simulink model "testtemp"  (Simulink 6.2)
settings: Solver=ode4  SolverMode=SingleTasking  StartTime=0  StopTime=0  MaxStep=10  RelTol=1e-3  AbsTol=1e-3
undefined symbols (not defined in the file or in its folder): d, n, pdelay, tgain, velreconsw
(part 1 of 3)
settings Model: Creator=jacobs  LastModifiedBy=jacobs  ExtModeAutoUpdateStatusClock=off
settings DataIOCC: LimitDataPoints=off  SaveOutput=off  SaveTime=off
settings OptimizationCC: BlockReduction=off  BooleanDataType=off
settings HardwareCC: TargetUnknown=on
settings STFCustomTargetCC: TargetFcnLib=ansi_tfl_tmw.mat  GenFloatMathFcnCalls=ANSI_C  ModelReferenceCompliant=off  SystemTargetFile=grt.tlc

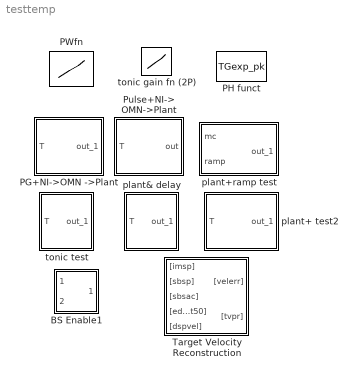
== system testtemp ==
  BS Enable1 : Subsystem
      mask Display: disp('FS\nEnab')
  PG+NI->OMN ->Plant : Subsystem
      mask Display: disp('PG+NI\n->OMN\n->Plant')
  PH funct : MATLABFcn  MATLABFcn=TGexp_pk
      mask Display: disp('Tonic\nGain')
  PWfn : Lookup  Orientation=down  InputValues=[ 0, 0.05:5, 5:10, 10:50 ]  OutputValues="[ 0, (0.05:5)*0+15,  (5:10)*1+10,  (10:50)*2]"  SaturateOnIntegerOverflow=on
  Pulse+NI-> OMN->Plant : Subsystem
      mask Display: disp('Pulse+NI\n->OMN\n->Plant')
  Target Velocity Reconstruction : Subsystem
      mask Display: disp('Target\nVelocity\nReconstruction')
  plant& delay : Subsystem
      mask Display: disp('plant &\ndelay')
  plant+ test2 : Subsystem
      mask Display: disp('PG->delay\n->plant')
  plant+ramp test : Subsystem
      mask Display: disp('plant+ramp\ntest')
  tonic gain fn (2P) : Lookup  InputValues=[ 0:90, 90:120 ]  OutputValues=[ (0:90)*( -.0039)+5.6, (90:120)*(-.0326)+8.18 ]  SaturateOnIntegerOverflow=on
  tonic test : Subsystem
      mask Display: disp('tonic\ntest')

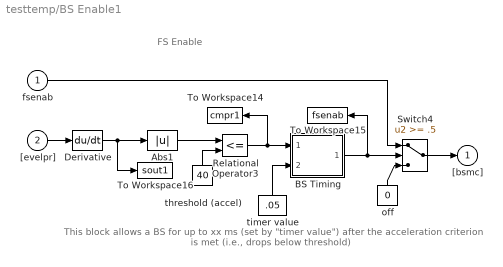
== system testtemp/BS Enable1 ==
  note: FS Enable
  note: This block allows a BS for up to xx ms (set by "timer value")
      | after the acceleration criterion is met (i.e., drops below threshold)
  fsenab : Inport  Port=1  LatchInput=off
  "[evelpr]" : Inport  Port=2  LatchInput=off
  Abs1 : Abs  SaturateOnIntegerOverflow=on
  BS Timing : Subsystem
      mask Display: disp('FS\nEnable\nTiming')
  Derivative : Derivative
      mask Display: disp('s')
  Relational Operator3 : RelationalOperator  Operator=<=  InputSameDT=on
  Switch4 : Switch  Threshold=.5  SaturateOnIntegerOverflow=on  InputSameDT=on
  To Workspace14 : ToWorkspace  VariableName=cmpr1  SaveFormat=Array
      settings: MaxDataPoints=10000
      mask Type: imsw1in
  To Workspace15 : ToWorkspace  VariableName=fsenab  SaveFormat=Array
      settings: MaxDataPoints=10000
      mask Type: imsw1in
  To Workspace16 : ToWorkspace  VariableName=sout1  SaveFormat=Array
      settings: MaxDataPoints=10000
      mask Type: imsw1in
  off : Constant  Orientation=up  Value=0
  threshold (accel) : Constant  Orientation=up  Value=40
  timer value : Constant  Orientation=up  Value=.05
  "[bsmc]" : Outport  InitialOutput=0
  wires:
  Relational Operator3/1 -> To Workspace14/1, BS Timing/1(From  <= [cmpr])
  Derivative/1 -> To Workspace16/1, Abs1/1
  Abs1/1 -> Relational Operator3/1
  BS Timing/1("[bsenab]") -> To Workspace15/1, Switch4/2
  "[evelpr]"/1 -> Derivative/1
  off/1 -> Switch4/3
  threshold (accel)/1 -> Relational Operator3/2
  fsenab/1 -> Switch4/1
  Switch4/1 -> "[bsmc]"/1
  timer value/1 -> BS Timing/2(timer dur)

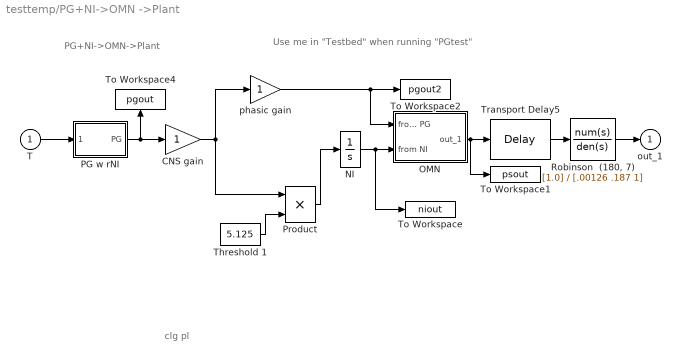
== system testtemp/PG+NI->OMN ->Plant ==
  note: clg
      | pl
  note: Use me in "Testbed" when running "PGtest"
  note: PG+NI->OMN->Plant
  T : Inport  Port=1  LatchInput=off
  CNS gain : Gain  SaturateOnIntegerOverflow=on
  NI : Integrator
  OMN : Subsystem
      mask Display: disp('<--"phasic"\nOMN\n<--"tonic"   ')
  PG w rNI : Subsystem
      mask Display: disp('PG rNI\n(2P)')
  Product : Product  SaturateOnIntegerOverflow=on  RndMeth=Zero  InputSameDT=on
  "Robinson  (180, 7)" : TransferFcn  Numerator=[1.0]  Denominator=[.00126 .187 1]
      mask Display: disp('2-pole')
  Threshold 1 : Constant  Value=5.125
  To Workspace : ToWorkspace  VariableName=niout  SaveFormat=Array
      settings: MaxDataPoints=10000
  To Workspace1 : ToWorkspace  VariableName=psout  SaveFormat=Array
      settings: MaxDataPoints=10000
  To Workspace2 : ToWorkspace  VariableName=pgout2  SaveFormat=Array
      settings: MaxDataPoints=10000
  To Workspace4 : ToWorkspace  VariableName=pgout  SaveFormat=Array
      settings: Orientation=up  MaxDataPoints=10000
  Transport Delay5 : TransportDelay  DelayTime=0.001
      mask Display: disp('"pdelay"\n(msec)')
  phasic gain : Gain  SaturateOnIntegerOverflow=on
  out_1 : Outport  InitialOutput=0
  wires:
  Threshold 1/1 -> Product/2
  PG w rNI/1(PG) -> CNS gain/1, To Workspace4/1
  Transport Delay5/1 -> "Robinson  (180, 7)"/1
  Product/1 -> NI/1
  "Robinson  (180, 7)"/1 -> out_1/1
  NI/1 -> OMN/2(from NI), To Workspace/1
  phasic gain/1 -> To Workspace2/1, OMN/1(from PG)
  OMN/1(out_1) -> Transport Delay5/1, To Workspace1/1
  CNS gain/1 -> phasic gain/1, Product/1
  T/1 -> PG w rNI/1(mcsprd)

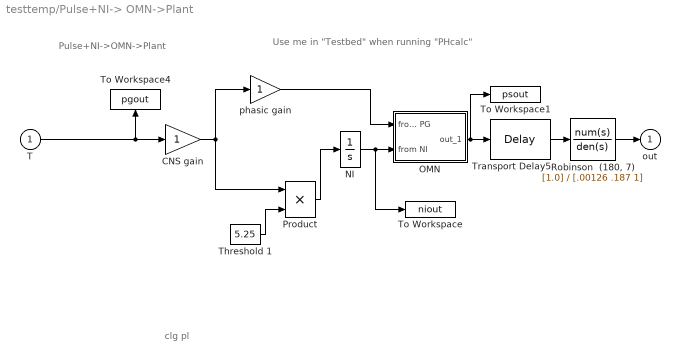
== system testtemp/Pulse+NI-> OMN->Plant ==
  note: clg
      | pl
  note: Use me in "Testbed" when running "PHcalc"
  note: Pulse+NI->OMN->Plant
  T : Inport  Port=1  LatchInput=off
  CNS gain : Gain  SaturateOnIntegerOverflow=on
  NI : Integrator
  OMN : Subsystem
      mask Display: disp('<--"phasic"\nOMN\n<--"tonic"   ')
  Product : Product  SaturateOnIntegerOverflow=on  RndMeth=Zero  InputSameDT=on
  "Robinson  (180, 7)" : TransferFcn  Numerator=[1.0]  Denominator=[.00126 .187 1]
      mask Display: disp('2-pole')
  Threshold 1 : Constant  Value=5.25
  To Workspace : ToWorkspace  VariableName=niout  SaveFormat=Array
      settings: MaxDataPoints=10000
  To Workspace1 : ToWorkspace  VariableName=psout  SaveFormat=Array
      settings: MaxDataPoints=10000
  To Workspace4 : ToWorkspace  VariableName=pgout  SaveFormat=Array
      settings: Orientation=up  MaxDataPoints=10000
  Transport Delay5 : TransportDelay  DelayTime=0.001
      mask Display: disp('"pdelay"\n(msec)')
  phasic gain : Gain  SaturateOnIntegerOverflow=on
  out : Outport  InitialOutput=0
  wires:
  Threshold 1/1 -> Product/2
  T/1 -> CNS gain/1, To Workspace4/1
  Transport Delay5/1 -> "Robinson  (180, 7)"/1
  Product/1 -> NI/1
  "Robinson  (180, 7)"/1 -> out/1
  NI/1 -> OMN/2(from NI), To Workspace/1
  phasic gain/1 -> OMN/1(from PG)
  OMN/1(out_1) -> Transport Delay5/1, To Workspace1/1
  CNS gain/1 -> phasic gain/1, Product/1

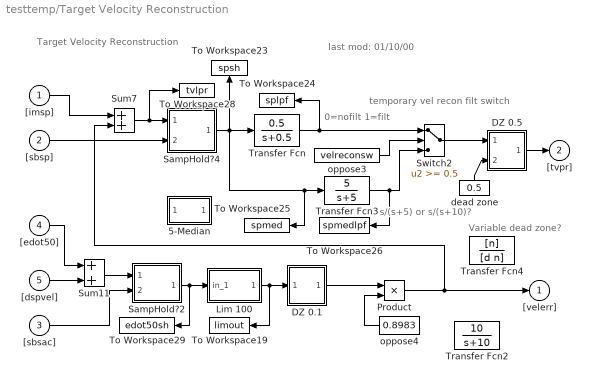
== system testtemp/Target Velocity Reconstruction ==
  note: last mod:
      | 01/10/00
  note: Target Velocity Reconstruction
  note: temporary
      | vel recon
      | filt switch
  note: 0=nofilt
      | 1=filt
  note: s/(s+5) or
      | s/(s+10)?
  note: Variable dead zone?
  "[imsp]" : Inport  Port=1  LatchInput=off
  "[sbsp]" : Inport  Port=2  LatchInput=off
  "[sbsac]" : Inport  Port=3  LatchInput=off
  "[edot50]" : Inport  Port=4  LatchInput=off
  "[dspvel]" : Inport  Port=5  LatchInput=off
  5-Median : Subsystem
      mask Display: disp('5-Med')
  DZ 0.1 : Subsystem
      mask Display: disp('Dead\nZone')
  DZ 0.5 : Subsystem
      mask Display: disp('Dead\nZone')
  Lim 100 : Subsystem
      mask Display: disp('Limiter')
  Product : Product  SaturateOnIntegerOverflow=on  RndMeth=Zero  InputSameDT=on
  SampHold?2 : Subsystem
      mask Display: disp('S=H\nH=L')
  SampHold?4 : Subsystem
      mask Display: disp('S=H\nH=L')
  Sum11 : Sum  SaturateOnIntegerOverflow=on  InputSameDT=on
  Sum7 : Sum  SaturateOnIntegerOverflow=on  InputSameDT=on
  Switch2 : Switch  Threshold=0.5  SaturateOnIntegerOverflow=on  InputSameDT=on
  To Workspace19 : ToWorkspace  VariableName=limout  SaveFormat=Array
      settings: MaxDataPoints=10000
  To Workspace23 : ToWorkspace  VariableName=spsh  SaveFormat=Array
      settings: Orientation=up  MaxDataPoints=10000
  To Workspace24 : ToWorkspace  VariableName=splpf  SaveFormat=Array
      settings: MaxDataPoints=10000
  To Workspace25 : ToWorkspace  VariableName=spmed  SaveFormat=Array
      settings: MaxDataPoints=10000
  To Workspace26 : ToWorkspace  VariableName=spmedlpf  SaveFormat=Array
      settings: MaxDataPoints=10000
  To Workspace28 : ToWorkspace  VariableName=tvlpr  SaveFormat=Array
      settings: MaxDataPoints=10000
  To Workspace29 : ToWorkspace  VariableName=edot50sh  SaveFormat=Array
      settings: MaxDataPoints=10000
  Transfer Fcn : TransferFcn  Numerator=[0.5]  Denominator=[1 0.5]
  Transfer Fcn2 : TransferFcn  Numerator=[10]  Denominator=[1 10]
  Transfer Fcn3 : TransferFcn  Numerator=[5]  Denominator=[1 5]
  Transfer Fcn4 : TransferFcn  Numerator=[n]  Denominator=[d n]
  dead zone : Constant  Orientation=up  Value=0.5
  oppose3 : Constant  Value=velreconsw
  oppose4 : Constant  Orientation=left  Value=0.8983
  "[velerr]" : Outport  InitialOutput=0
  "[tvpr]" : Outport  Port=2  InitialOutput=0
  wires:
  "[sbsp]"/1 -> SampHold?4/2(S/H?)
  SampHold?4/1(output) -> Transfer Fcn/1, To Workspace23/1, To Workspace25/1, Transfer Fcn3/1
  "[imsp]"/1 -> Sum7/1
  Sum7/1 -> SampHold?4/1(Input), To Workspace28/1
  Transfer Fcn/1 -> To Workspace24/1, Switch2/1
  oppose3/1 -> Switch2/2
  Switch2/1 -> DZ 0.5/1(in_1)
  "[sbsac]"/1 -> SampHold?2/2(S/H?)
  "[dspvel]"/1 -> Sum11/2
  "[edot50]"/1 -> Sum11/1
  Sum11/1 -> SampHold?2/1(Input)
  Lim 100/1(out_1) -> To Workspace19/1, DZ 0.1/1(in_1)
  SampHold?2/1(output) -> To Workspace29/1, Lim 100/1(in_1)
  DZ 0.1/1(out_1) -> Product/1
  Product/1 -> Sum7/2, "[velerr]"/1
  oppose4/1 -> Product/2
  DZ 0.5/1(out_1) -> "[tvpr]"/1
  dead zone/1 -> DZ 0.5/2(in_2)
  Transfer Fcn3/1 -> Switch2/3, To Workspace26/1

== system testtemp/plant& delay ==
  note: clg
      | pl
  note: Use me in "Testbed" when running "PHcalc"
  T : Inport  Port=1  LatchInput=off
  "Robinson  (180, 7)" : TransferFcn  Numerator=[1.0]  Denominator=[.00126 .187 1]
      mask Display: disp('2-pole')
  Transport Delay5 : TransportDelay  DelayTime=pdelay
      mask Display: disp('"pdelay"\n(ms)')
  out_1 : Outport  InitialOutput=0
  wires:
  "Robinson  (180, 7)"/1 -> out_1/1
  T/1 -> Transport Delay5/1
  Transport Delay5/1 -> "Robinson  (180, 7)"/1

== system testtemp/plant+ test2 ==
  note: clg
      | pl
  note: PG->delay->Plant
  T : Inport  Port=1  LatchInput=off
  PG w rNI : Subsystem
      mask Display: disp('PG rNI\n(2P)')
  "Robinson  (180, 7)" : TransferFcn  Numerator=[1.0]  Denominator=[.00126 .187 1]
      mask Display: disp('2-pole')
  To Workspace4 : ToWorkspace  VariableName=pgout  SaveFormat=Array
      settings: Orientation=up  MaxDataPoints=10000
  Transport Delay5 : TransportDelay  DelayTime=0.01
      mask Display: disp('"pdelay"\n(msec)')
  Transport Delay6 : TransportDelay  DelayTime=0.01
      mask Display: disp('"pdelay"\n(msec)')
  out_1 : Outport  InitialOutput=0
  wires:
  PG w rNI/1(PG) -> Transport Delay5/1, To Workspace4/1
  Transport Delay5/1 -> "Robinson  (180, 7)"/1
  Transport Delay6/1 -> out_1/1
  "Robinson  (180, 7)"/1 -> Transport Delay6/1
  T/1 -> PG w rNI/1(mcsprd)

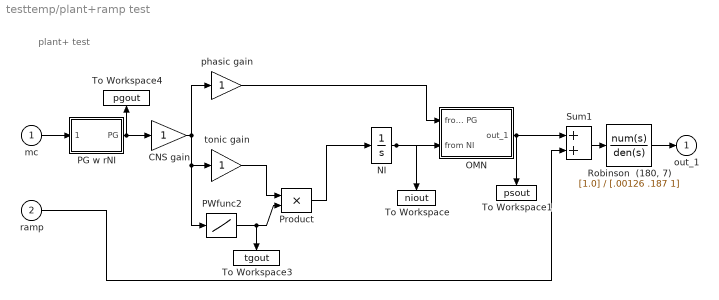
== system testtemp/plant+ramp test ==
  note: plant+ test
  mc : Inport  Port=1  LatchInput=off
  ramp : Inport  Port=2  LatchInput=off
  CNS gain : Gain  SaturateOnIntegerOverflow=on
  NI : Integrator
  OMN : Subsystem
      mask Display: disp('<--"phasic"\nOMN\n<--"tonic"   ')
  PG w rNI : Subsystem
      mask Display: disp('PG rNI\n(2P)')
  PWfunc2 : Lookup  InputValues=[ 0:90, 91:120 ]  OutputValues=[ (0:90)*( -.0039)+5.6, (91:120)*(-.0326)+8.18 ]  SaturateOnIntegerOverflow=on
  Product : Product  SaturateOnIntegerOverflow=on  RndMeth=Zero  InputSameDT=on
  "Robinson  (180, 7)" : TransferFcn  Numerator=[1.0]  Denominator=[.00126 .187 1]
      mask Display: disp('2-pole')
  Sum1 : Sum  SaturateOnIntegerOverflow=on  InputSameDT=on
  To Workspace : ToWorkspace  VariableName=niout  SaveFormat=Array
      settings: Orientation=down  MaxDataPoints=10000
  To Workspace1 : ToWorkspace  VariableName=psout  SaveFormat=Array
      settings: Orientation=down  MaxDataPoints=10000
  To Workspace3 : ToWorkspace  VariableName=tgout  SaveFormat=Array
      settings: Orientation=down  MaxDataPoints=10000
  To Workspace4 : ToWorkspace  VariableName=pgout  SaveFormat=Array
      settings: Orientation=up  MaxDataPoints=10000
  phasic gain : Gain  SaturateOnIntegerOverflow=on
  tonic gain : Gain  SaturateOnIntegerOverflow=on
  out_1 : Outport  InitialOutput=0
  wires:
  ramp/1 -> Sum1/2
  Sum1/1 -> "Robinson  (180, 7)"/1
  Product/1 -> NI/1
  PWfunc2/1 -> Product/2, To Workspace3/1
  mc/1 -> PG w rNI/1(mcsprd)
  tonic gain/1 -> Product/1
  PG w rNI/1(PG) -> CNS gain/1, To Workspace4/1
  "Robinson  (180, 7)"/1 -> out_1/1
  NI/1 -> To Workspace/1, OMN/2(from NI)
  phasic gain/1 -> OMN/1(from PG)
  CNS gain/1 -> tonic gain/1, PWfunc2/1, phasic gain/1
  OMN/1(out_1) -> To Workspace1/1, Sum1/1

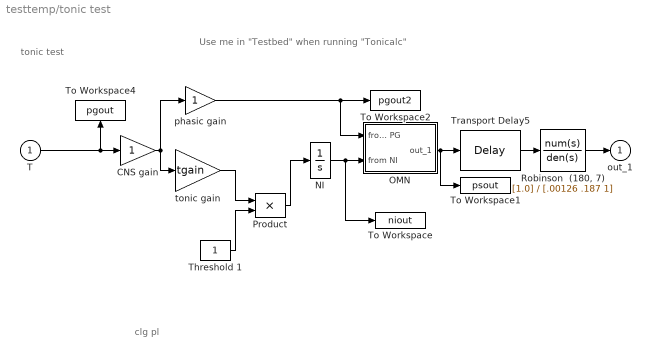
== system testtemp/tonic test ==
  note: clg
      | pl
  note: Use me in "Testbed" when running "Tonicalc"
  note: tonic test
  T : Inport  Port=1  LatchInput=off
  CNS gain : Gain  SaturateOnIntegerOverflow=on
  NI : Integrator
  OMN : Subsystem
      mask Display: disp('<--"phasic"\nOMN\n<--"tonic"   ')
  Product : Product  SaturateOnIntegerOverflow=on  RndMeth=Zero  InputSameDT=on
  "Robinson  (180, 7)" : TransferFcn  Numerator=[1.0]  Denominator=[.00126 .187 1]
      mask Display: disp('2-pole')
  Threshold 1 : Constant
  To Workspace : ToWorkspace  VariableName=niout  SaveFormat=Array
      settings: MaxDataPoints=10000
  To Workspace1 : ToWorkspace  VariableName=psout  SaveFormat=Array
      settings: MaxDataPoints=10000
  To Workspace2 : ToWorkspace  VariableName=pgout2  SaveFormat=Array
      settings: MaxDataPoints=10000
  To Workspace4 : ToWorkspace  VariableName=pgout  SaveFormat=Array
      settings: Orientation=up  MaxDataPoints=10000
  Transport Delay5 : TransportDelay  DelayTime=0.001
      mask Display: disp('"pdelay"\n(msec)')
  phasic gain : Gain  SaturateOnIntegerOverflow=on
  tonic gain : Gain  Gain=tgain  SaturateOnIntegerOverflow=on
  out_1 : Outport  InitialOutput=0
  wires:
  Transport Delay5/1 -> "Robinson  (180, 7)"/1
  Product/1 -> NI/1
  Threshold 1/1 -> Product/2
  tonic gain/1 -> Product/1
  T/1 -> CNS gain/1, To Workspace4/1
  "Robinson  (180, 7)"/1 -> out_1/1
  NI/1 -> OMN/2(from NI), To Workspace/1
  phasic gain/1 -> To Workspace2/1, OMN/1(from PG)
  CNS gain/1 -> tonic gain/1, phasic gain/1
  OMN/1(out_1) -> Transport Delay5/1, To Workspace1/1

== system testtemp/BS Enable1/BS Timing ==
  note: (FF init state: Q=0)
  note: * Leading Edge of input ENABLEs output
  note: Operation:
  note: *BS Enabling is initially DISABLED
  note: * Output of TIMER circuit DISABLES output
  note: BS Timing
  From  <= [cmpr] : Inport  Port=1  LatchInput=off
  timer dur : Inport  Orientation=up  Port=2  LatchInput=off
  Latch1 : Subsystem  mask(Latch){@1=0}
      mask prompts: @1 "Initial State for Output "Q":"
      mask help: Latch
      mask init:
      | ini=(@1~=0);
      mask Help: Latches the S input.  When S (set) is one, the Q output  becomes one.  The output remains one until the R (reset) input becomes one, forcing the output to zero.  If both R and S are one, the latch will be in an undefined state.
      mask Display: disp('S   Q\n\nR  !Q')
  event timer2 : Subsystem
      mask Display: disp('Event\nTimer2')
  leading edge detect : Subsystem
      mask Display: disp('Leading\nEdge Det')
  "[bsenab]" : Outport  InitialOutput=0
  wires:
  From  <= [cmpr]/1 -> leading edge detect/1(in_1), event timer2/1(_PG)
  leading edge detect/1(out_1) -> Latch1/1(in_1)
  event timer2/1(out_1) -> Latch1/2(in_2)
  Latch1/1(out_1) -> "[bsenab]"/1
  timer dur/1 -> event timer2/2(_timer value (port))

== system testtemp/PG+NI->OMN ->Plant/OMN ==
  note: Note that the OMN properly combines the pulse with the output of the NI, by latching
      | that output to its value at the moment the pulse appears.
  note: OMN
  note: Operation: when the pulse is active ("from PG") it activates the switch, passing the
      | upper input through to the output.  When the pulse is over, the switch changes,
      | allowing the lower input (from the NI) to pass.
  note: This block behaves like the ocular motor neurons,combining a phasic pulse (from PG)
      | with the tonic step produced by integration of the step, yielding a Pulse-Step
      | to drive the plant.
  from PG : Inport  Port=1  LatchInput=off
  from NI : Inport  Port=2  LatchInput=off
  Abs : Abs  SaturateOnIntegerOverflow=on
  Gain _ : Gain  Gain=1.0  SaturateOnIntegerOverflow=on
  SampHold? : Subsystem
      mask Display: disp('S&H\n(L)')
  Sign : Subsystem
      mask Type: Sign
      mask Description: y = sign(x)
      mask Help: Sign Function:\n\t\t\ty = 1 if x > 0\n\t\t\ty = 0 if x = 0\n\t\t\ty = -1 if x < 0
      mask Display: plot(-50,-50,50,50,[-50,50],[0,0],[0,0],[-50,50],[-40,0],[-30,-30],[0,40],[30,30])
  Sum : Sum  SaturateOnIntegerOverflow=on  InputSameDT=on
  Switch : Switch  Threshold=.5  SaturateOnIntegerOverflow=on  InputSameDT=on
  To Workspace : ToWorkspace  VariableName=ni_in  SaveFormat=Array
      settings: MaxDataPoints=10000
  To Workspace1 : ToWorkspace  VariableName=pg_in  SaveFormat=Array
      settings: MaxDataPoints=10000
  out_1 : Outport  InitialOutput=0
  wires:
  SampHold?/1(output) -> Sum/2
  Sign/1(out_1) -> Switch/2, SampHold?/2(S/H?)
  from PG/1 -> Abs/1, Gain _/1
  Sum/1 -> Switch/1, To Workspace1/1
  from NI/1 -> Switch/3, To Workspace/1, SampHold?/1(Input)
  Gain _/1 -> Sum/1
  Switch/1 -> out_1/1
  Abs/1 -> Sign/1(in_1)

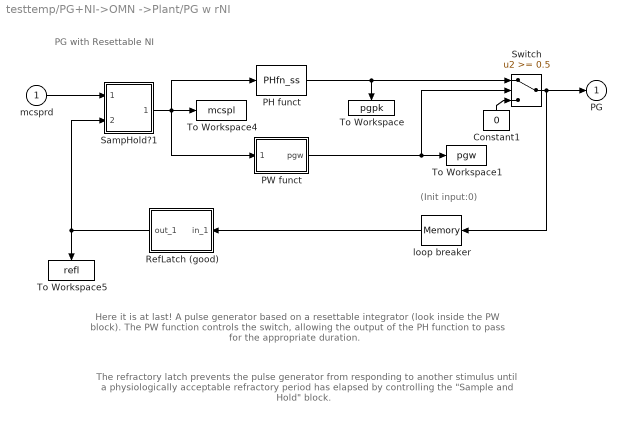
== system testtemp/PG+NI->OMN ->Plant/PG w rNI ==
  note: (Init input:0)
  note: PG with Resettable NI
  note: The refractory latch prevents the pulse generator from responding to another stimulus until a
      | physiologically acceptable refractory period has elapsed by controlling the "Sample and Hold" block.
  note: Here it is at last!  A pulse generator based on a resettable integrator (look inside the PW
      | block).  The PW function controls the switch, allowing the output of the PH function to pass
      | for the appropriate duration.
  mcsprd : Inport  Port=1  LatchInput=off
  Constant1 : Constant  Orientation=up  Value=0
  PH funct : MATLABFcn  MATLABFcn=PHfn_ss
      mask Display: disp('PH\nfunction')
  PW funct : Subsystem
      mask Display: disp('PW\nfunction')
  RefLatch (good) : Subsystem  Orientation=left  mask{@1=50}
      mask prompts: @1 "Refractory Period (ms)"
      mask help: Refractory Latch
      mask init:
      | delay=@1;
      mask Display: disp('Refract\nLatch')
  SampHold?1 : Subsystem
      mask Display: disp('S&H\n(S=H)\n(H=L)')
  Switch : Switch  Threshold=0.5  SaturateOnIntegerOverflow=on  InputSameDT=on
  To Workspace : ToWorkspace  VariableName=pgpk  SaveFormat=Array
      settings: Orientation=down  MaxDataPoints=10000
  To Workspace1 : ToWorkspace  VariableName=pgw  SaveFormat=Array
      settings: MaxDataPoints=10000
  To Workspace4 : ToWorkspace  VariableName=mcspl  SaveFormat=Array
      settings: MaxDataPoints=10000
  To Workspace5 : ToWorkspace  VariableName=refl  SaveFormat=Array
      settings: Orientation=down  MaxDataPoints=10000
  loop breaker : Memory  Orientation=left
  PG : Outport  InitialOutput=0
  wires:
  SampHold?1/1(output) -> PH funct/1, PW funct/1(mcspl), To Workspace4/1
  RefLatch (good)/1(out_1) -> SampHold?1/2(S/H?), To Workspace5/1
  loop breaker/1 -> RefLatch (good)/1(in_1)
  Constant1/1 -> Switch/3
  mcsprd/1 -> SampHold?1/1(Input)
  Switch/1 -> PG/1, loop breaker/1
  PW funct/1(pgw) -> Switch/2, To Workspace1/1
  PH funct/1 -> Switch/1, To Workspace/1

== system testtemp/Pulse+NI-> OMN->Plant/OMN ==
  note: Note that the OMN properly combines the pulse with the output of the NI, by latching
      | that output to its value at the moment the pulse appears.
  note: OMN
  note: Operation: when the pulse is active ("from PG") it activates the switch, passing the
      | upper input through to the output.  When the pulse is over, the switch changes,
      | allowing the lower input (from the NI) to pass.
  note: This block behaves like the ocular motor neurons,combining a phasic pulse (from PG)
      | with the tonic step produced by integration of the step, yielding a Pulse-Step
      | to drive the plant.
  from PG : Inport  Port=1  LatchInput=off
  from NI : Inport  Port=2  LatchInput=off
  Abs : Abs  SaturateOnIntegerOverflow=on
  Gain _ : Gain  Gain=1.0  SaturateOnIntegerOverflow=on
  SampHold? : Subsystem
      mask Display: disp('S&H\n(L)')
  Sign : Subsystem
      mask Type: Sign
      mask Description: y = sign(x)
      mask Help: Sign Function:\n\t\t\ty = 1 if x > 0\n\t\t\ty = 0 if x = 0\n\t\t\ty = -1 if x < 0
      mask Display: plot(-50,-50,50,50,[-50,50],[0,0],[0,0],[-50,50],[-40,0],[-30,-30],[0,40],[30,30])
  Sum : Sum  SaturateOnIntegerOverflow=on  InputSameDT=on
  Switch : Switch  Threshold=.5  SaturateOnIntegerOverflow=on  InputSameDT=on
  To Workspace : ToWorkspace  VariableName=ni_in  SaveFormat=Array
      settings: MaxDataPoints=10000
  To Workspace1 : ToWorkspace  VariableName=pg_in  SaveFormat=Array
      settings: MaxDataPoints=10000
  out_1 : Outport  InitialOutput=0
  wires:
  SampHold?/1(output) -> Sum/2
  Sign/1(out_1) -> Switch/2, SampHold?/2(S/H?)
  from PG/1 -> Abs/1, Gain _/1
  Sum/1 -> Switch/1, To Workspace1/1
  from NI/1 -> Switch/3, To Workspace/1, SampHold?/1(Input)
  Gain _/1 -> Sum/1
  Switch/1 -> out_1/1
  Abs/1 -> Sign/1(in_1)

== system testtemp/Target Velocity Reconstruction/5-Median ==
  note: 5-pt median filter
  in_1 : Inport  Port=1  LatchInput=off
  MATLAB Fcn : MATLABFcn  MATLABFcn=median  OutputDimensions=1
      mask Display: disp('Median')
  Memory{,1..3} (4 alike) : Memory
  Mux : Mux  Orientation=down  Inputs=5
  out_1 : Outport  InitialOutput=0
  wires:
  Mux/1 -> MATLAB Fcn/1
  in_1/1 -> Mux/1, Memory1/1
  Memory/1 -> Mux/3, Memory2/1
  Memory2/1 -> Mux/4, Memory3/1
  Memory3/1 -> Mux/5
  Memory1/1 -> Mux/2, Memory/1
  MATLAB Fcn/1 -> out_1/1

== system testtemp/Target Velocity Reconstruction/DZ 0.1 ==
  note: We just output zero when the dead zone is in effect, and leave the
      |  output alone the rest of the time.
  note: This block is a better implementation of a dead zone than  the
      | block supplied by SIMULINK, because here we don't _subtract_
      | the dead zone from the rest of output.
  in_1 : Inport  Port=1  LatchInput=off
  Abs : Abs  Orientation=down  SaturateOnIntegerOverflow=on
  Relational Operator : RelationalOperator  InputSameDT=on
  Switch6 : Switch  Threshold=.5  SaturateOnIntegerOverflow=on  InputSameDT=on
  dead zone : Constant  Orientation=up  Value=.1
  pos (deg) criterion1 : Constant  Orientation=left  Value=0
  out_1 : Outport  InitialOutput=0
  wires:
  Relational Operator/1 -> Switch6/2
  dead zone/1 -> Relational Operator/2
  pos (deg) criterion1/1 -> Switch6/3
  Abs/1 -> Relational Operator/1
  in_1/1 -> Abs/1, Switch6/1
  Switch6/1 -> out_1/1

== system testtemp/Target Velocity Reconstruction/DZ 0.5 ==
  note: We just output zero when the dead zone is in effect, and leave the
      |  output alone the rest of the time.
  note: This block is a better implementation of a dead zone than  the
      | block supplied by SIMULINK, because here we don't _subtract_
      | the dead zone from the rest of output.
  in_1 : Inport  Port=1  LatchInput=off
  in_2 : Inport  Port=2  LatchInput=off
  Abs : Abs  Orientation=down  SaturateOnIntegerOverflow=on
  Relational Operator : RelationalOperator  InputSameDT=on
  Switch6 : Switch  Threshold=.5  SaturateOnIntegerOverflow=on  InputSameDT=on
  pos (deg) criterion1 : Constant  Orientation=left  Value=0
  out_1 : Outport  InitialOutput=0
  wires:
  Relational Operator/1 -> Switch6/2
  pos (deg) criterion1/1 -> Switch6/3
  Abs/1 -> Relational Operator/1
  in_1/1 -> Abs/1, Switch6/1
  Switch6/1 -> out_1/1
  in_2/1 -> Relational Operator/2

== system testtemp/Target Velocity Reconstruction/Lim 100 ==
  note: This block limits outputs to less than or equal to the "Limit" constant.
      | Inputs greater than "Limit" yield a zero output.
  in_1 : Inport  Port=1  LatchInput=off
  Abs : Abs  SaturateOnIntegerOverflow=on
  Limit : Constant  Orientation=up  Value=100
  Product : Product  SaturateOnIntegerOverflow=on  RndMeth=Zero  InputSameDT=on
  Relational Operator : RelationalOperator  Operator=<=  InputSameDT=on
  out_1 : Outport  InitialOutput=0
  wires:
  in_1/1 -> Product/1, Abs/1
  Abs/1 -> Relational Operator/1
  Relational Operator/1 -> Product/2
  Limit/1 -> Relational Operator/2
  Product/1 -> out_1/1

== system testtemp/Target Velocity Reconstruction/SampHold?2 ==
  note: When "S/H?" is HIGH, then "Input" is switched directly to the
      | output ("sample").  When "S/H?" is LOW, the current output is
      | maintained ("hold").
  Input : Inport  Port=1  LatchInput=off
  S/H? : Inport  Port=2  LatchInput=off
  Memory : Memory  Orientation=left
  Sign : Subsystem
      mask Type: Sign
      mask Description: y = sign(x)
      mask Help: Sign Function:\n\t\t\ty = 1 if x > 0\n\t\t\ty = 0 if x = 0\n\t\t\ty = -1 if x < 0
      mask Display: plot(-50,-50,50,50,[-50,50],[0,0],[0,0],[-50,50],[-40,0],[-30,-30],[0,40],[30,30])
  Switch2 : Switch  Threshold=0.5  SaturateOnIntegerOverflow=on  InputSameDT=on
  output : Outport  InitialOutput=0
  wires:
  Memory/1 -> Switch2/3
  Input/1 -> Switch2/1
  Switch2/1 -> Memory/1, output/1
  Sign/1(out_1) -> Switch2/2
  S/H?/1 -> Sign/1(in_1)

== system testtemp/Target Velocity Reconstruction/SampHold?4 ==
  note: When "S/H?" is HIGH, then "Input" is switched directly to the
      | output ("sample").  When "S/H?" is LOW, the current output is
      | maintained ("hold").
  Input : Inport  Port=1  LatchInput=off
  S/H? : Inport  Port=2  LatchInput=off
  Memory : Memory  Orientation=left
  Sign : Subsystem
      mask Type: Sign
      mask Description: y = sign(x)
      mask Help: Sign Function:\n\t\t\ty = 1 if x > 0\n\t\t\ty = 0 if x = 0\n\t\t\ty = -1 if x < 0
      mask Display: plot(-50,-50,50,50,[-50,50],[0,0],[0,0],[-50,50],[-40,0],[-30,-30],[0,40],[30,30])
  Switch2 : Switch  Threshold=0.5  SaturateOnIntegerOverflow=on  InputSameDT=on
  output : Outport  InitialOutput=0
  wires:
  S/H?/1 -> Sign/1(in_1)
  Sign/1(out_1) -> Switch2/2
  Switch2/1 -> output/1, Memory/1
  Input/1 -> Switch2/1
  Memory/1 -> Switch2/3

== system testtemp/plant+ test2/PG w rNI ==
  note: (Init input:0)
  note: PG with Resettable NI
  note: The refractory latch prevents the pulse generator from responding to another stimulus until a
      | physiologically acceptable refractory period has elapsed by controlling the "Sample and Hold" block.
  note: Here it is at last!  A pulse generator based on a resettable integrator (look inside the PW
      | block).  The PW function controls the switch, allowing the output of the PH function to pass
      | for the appropriate duration.
  mcsprd : Inport  Port=1  LatchInput=off
  Constant1 : Constant  Orientation=up  Value=0
  PH funct : MATLABFcn  MATLABFcn=PHfn_ss
      mask Display: disp('PH\nfunction')
  PW funct : Subsystem
      mask Display: disp('PW\nfunction')
  RefLatch (good) : Subsystem  Orientation=left  mask{@1=50}
      mask prompts: @1 "Refractory Period (ms)"
      mask help: Refractory Latch
      mask init:
      | delay=@1;
      mask Display: disp('Refract\nLatch')
  SampHold?1 : Subsystem
      mask Display: disp('S&H\n(S=H)\n(H=L)')
  Switch : Switch  Threshold=0.5  SaturateOnIntegerOverflow=on  InputSameDT=on
  To Workspace : ToWorkspace  VariableName=pgpk  SaveFormat=Array
      settings: Orientation=down  MaxDataPoints=10000
  To Workspace1 : ToWorkspace  VariableName=pgw  SaveFormat=Array
      settings: MaxDataPoints=10000
  To Workspace4 : ToWorkspace  VariableName=mcspl  SaveFormat=Array
      settings: MaxDataPoints=10000
  To Workspace5 : ToWorkspace  VariableName=refl  SaveFormat=Array
      settings: Orientation=down  MaxDataPoints=10000
  loop breaker : Memory  Orientation=left
  PG : Outport  InitialOutput=0
  wires:
  SampHold?1/1(output) -> PH funct/1, PW funct/1(mcspl), To Workspace4/1
  RefLatch (good)/1(out_1) -> SampHold?1/2(S/H?), To Workspace5/1
  loop breaker/1 -> RefLatch (good)/1(in_1)
  Constant1/1 -> Switch/3
  mcsprd/1 -> SampHold?1/1(Input)
  Switch/1 -> PG/1, loop breaker/1
  PW funct/1(pgw) -> Switch/2, To Workspace1/1
  PH funct/1 -> Switch/1, To Workspace/1

== system testtemp/plant+ramp test/OMN ==
  note: Note that the OMN properly combines the pulse with the output of the NI, by latching
      | that output to its value at the moment the pulse appears.
  note: OMN
  note: Operation: when the pulse is active ("from PG") it activates the switch, passing the
      | upper input through to the output.  When the pulse is over, the switch changes,
      | allowing the lower input (from the NI) to pass.
  note: This block behaves like the ocular motor neurons,combining a phasic pulse (from PG)
      | with the tonic step produced by integration of the step, yielding a Pulse-Step
      | to drive the plant.
  from PG : Inport  Port=1  LatchInput=off
  from NI : Inport  Port=2  LatchInput=off
  Abs : Abs  SaturateOnIntegerOverflow=on
  Gain _ : Gain  Gain=1.0  SaturateOnIntegerOverflow=on
  SampHold? : Subsystem
      mask Display: disp('S&H\n(L)')
  Sign : Subsystem
      mask Type: Sign
      mask Description: y = sign(x)
      mask Help: Sign Function:\n\t\t\ty = 1 if x > 0\n\t\t\ty = 0 if x = 0\n\t\t\ty = -1 if x < 0
      mask Display: plot(-50,-50,50,50,[-50,50],[0,0],[0,0],[-50,50],[-40,0],[-30,-30],[0,40],[30,30])
  Sum : Sum  SaturateOnIntegerOverflow=on  InputSameDT=on
  Switch : Switch  Threshold=.5  SaturateOnIntegerOverflow=on  InputSameDT=on
  To Workspace : ToWorkspace  VariableName=ni_in  SaveFormat=Array
      settings: MaxDataPoints=10000
  To Workspace1 : ToWorkspace  VariableName=pg_in  SaveFormat=Array
      settings: MaxDataPoints=10000
  out_1 : Outport  InitialOutput=0
  wires:
  SampHold?/1(output) -> Sum/2
  Sign/1(out_1) -> Switch/2, SampHold?/2(S/H?)
  from PG/1 -> Abs/1, Gain _/1
  Sum/1 -> Switch/1, To Workspace1/1
  from NI/1 -> Switch/3, To Workspace/1, SampHold?/1(Input)
  Gain _/1 -> Sum/1
  Switch/1 -> out_1/1
  Abs/1 -> Sign/1(in_1)

== system testtemp/plant+ramp test/PG w rNI ==
  note: (Init input:0)
  note: PG with Resettable NI
  note: The refractory latch prevents the pulse generator from responding to another stimulus until a
      | physiologically acceptable refractory period has elapsed by controlling the "Sample and Hold" block.
  note: Here it is at last!  A pulse generator based on a resettable integrator (look inside the PW
      | block).  The PW function controls the switch, allowing the output of the PH function to pass
      | for the appropriate duration.
  mcsprd : Inport  Port=1  LatchInput=off
  Constant1 : Constant  Orientation=up  Value=0
  PH funct : MATLABFcn  MATLABFcn=PHfn_ss
      mask Display: disp('PH\nfunction')
  PW funct : Subsystem
      mask Display: disp('PW\nfunction')
  RefLatch (good) : Subsystem  Orientation=left  mask{@1=50}
      mask prompts: @1 "Refractory Period (ms)"
      mask help: Refractory Latch
      mask init:
      | delay=@1;
      mask Display: disp('Refract\nLatch')
  SampHold?1 : Subsystem
      mask Display: disp('S&H\n(S=H)\n(H=L)')
  Switch : Switch  Threshold=0.5  SaturateOnIntegerOverflow=on  InputSameDT=on
  To Workspace : ToWorkspace  VariableName=pgpk  SaveFormat=Array
      settings: Orientation=down  MaxDataPoints=10000
  To Workspace1 : ToWorkspace  VariableName=pgw  SaveFormat=Array
      settings: MaxDataPoints=10000
  To Workspace4 : ToWorkspace  VariableName=mcspl  SaveFormat=Array
      settings: MaxDataPoints=10000
  To Workspace5 : ToWorkspace  VariableName=refl  SaveFormat=Array
      settings: Orientation=down  MaxDataPoints=10000
  loop breaker : Memory  Orientation=left
  PG : Outport  InitialOutput=0
  wires:
  SampHold?1/1(output) -> PH funct/1, PW funct/1(mcspl), To Workspace4/1
  RefLatch (good)/1(out_1) -> SampHold?1/2(S/H?), To Workspace5/1
  loop breaker/1 -> RefLatch (good)/1(in_1)
  Constant1/1 -> Switch/3
  mcsprd/1 -> SampHold?1/1(Input)
  Switch/1 -> PG/1, loop breaker/1
  PW funct/1(pgw) -> Switch/2, To Workspace1/1
  PH funct/1 -> Switch/1, To Workspace/1

== system testtemp/tonic test/OMN ==
  note: Note that the OMN properly combines the pulse with the output of the NI, by latching
      | that output to its value at the moment the pulse appears.
  note: OMN
  note: Operation: when the pulse is active ("from PG") it activates the switch, passing the
      | upper input through to the output.  When the pulse is over, the switch changes,
      | allowing the lower input (from the NI) to pass.
  note: This block behaves like the ocular motor neurons,combining a phasic pulse (from PG)
      | with the tonic step produced by integration of the step, yielding a Pulse-Step
      | to drive the plant.
  from PG : Inport  Port=1  LatchInput=off
  from NI : Inport  Port=2  LatchInput=off
  Abs : Abs  SaturateOnIntegerOverflow=on
  Gain _ : Gain  Gain=1.0  SaturateOnIntegerOverflow=on
  SampHold? : Subsystem
      mask Display: disp('S&H\n(L)')
  Sign : Subsystem
      mask Type: Sign
      mask Description: y = sign(x)
      mask Help: Sign Function:\n\t\t\ty = 1 if x > 0\n\t\t\ty = 0 if x = 0\n\t\t\ty = -1 if x < 0
      mask Display: plot(-50,-50,50,50,[-50,50],[0,0],[0,0],[-50,50],[-40,0],[-30,-30],[0,40],[30,30])
  Sum : Sum  SaturateOnIntegerOverflow=on  InputSameDT=on
  Switch : Switch  Threshold=.5  SaturateOnIntegerOverflow=on  InputSameDT=on
  To Workspace : ToWorkspace  VariableName=ni_in  SaveFormat=Array
      settings: MaxDataPoints=10000
  To Workspace1 : ToWorkspace  VariableName=pg_in  SaveFormat=Array
      settings: MaxDataPoints=10000
  out_1 : Outport  InitialOutput=0
  wires:
  SampHold?/1(output) -> Sum/2
  Sign/1(out_1) -> Switch/2, SampHold?/2(S/H?)
  from PG/1 -> Abs/1, Gain _/1
  Sum/1 -> Switch/1, To Workspace1/1
  from NI/1 -> Switch/3, To Workspace/1, SampHold?/1(Input)
  Gain _/1 -> Sum/1
  Switch/1 -> out_1/1
  Abs/1 -> Sign/1(in_1)

== system testtemp/BS Enable1/BS Timing/Latch1 ==
  in_1 : Inport  Port=1  LatchInput=off
  in_2 : Inport  Port=2  LatchInput=off
  Demux : Demux  Outputs=2
  Logic : CombinatorialLogic  TruthTable=[0 1;0 1;1 0;0 1;1 0;0 1;1 0;1 0]
  Memory : Memory  Orientation=left  X0=ini
  Mux : Mux  Inputs=3
  out_1 : Outport  InitialOutput=0
  out_2 : Outport  Port=2  InitialOutput=0
  wires:
  in_2/1 -> Mux/3
  in_1/1 -> Mux/2
  Memory/1 -> Mux/1
  Demux/1 -> Memory/1, out_1/1
  Mux/1 -> Logic/1
  Logic/1 -> Demux/1
  Demux/2 -> out_2/1

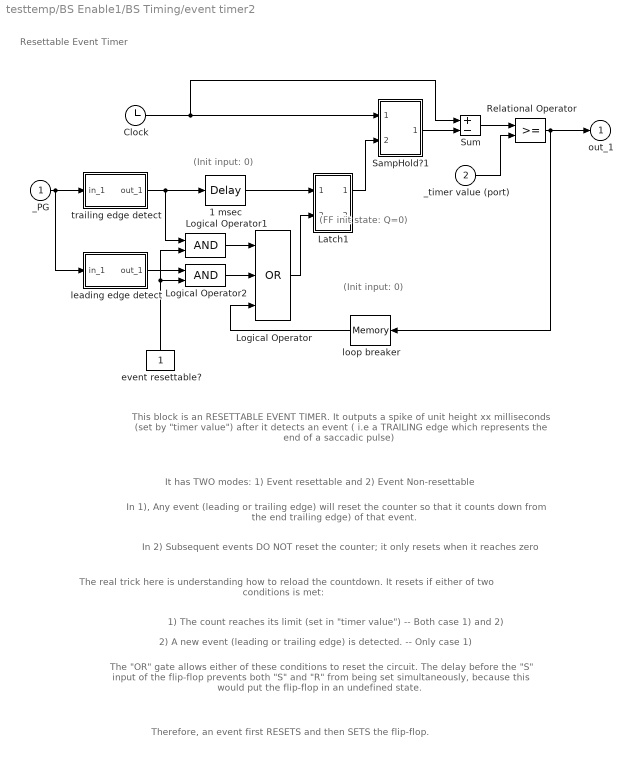
== system testtemp/BS Enable1/BS Timing/event timer2 ==
  note: In 2) Subsequent events DO NOT reset the counter; it only resets when it
      | reaches zero
  note: 2) A new event (leading or trailing edge) is detected. -- Only case 1)
  note: 1) The count reaches its limit (set in "timer value") -- Both case 1) and 2)
  note: In 1), Any event (leading or trailing edge) will reset the counter so that it
      | counts down from the end trailing edge) of that event.
  note: It has TWO modes: 1) Event resettable and 2) Event Non-resettable
  note: The real trick here is understanding how to reload the countdown.
      | It resets if either of two conditions is met:
  note: The "OR" gate allows either of these conditions to reset the circuit.  The delay before the
      | "S" input of the flip-flop prevents both "S" and "R" from being set simultaneously, because
      | this would put the flip-flop in an undefined state.
  note: Therefore, an event first RESETS and then SETS the flip-flop.
  note: (Init input: 0)
  note: (FF init state: Q=0)
  note: (Init input: 0)
  note: This block is an RESETTABLE EVENT TIMER.  It outputs a spike of unit height xx milliseconds
      | (set by "timer value") after it detects an event ( i.e a TRAILING edge which represents the end of a
      |  saccadic pulse)
  note: Resettable
      | Event Timer
  _PG : Inport  Port=1  LatchInput=off
  _timer value (port) : Inport  Port=2  LatchInput=off
  1 msec : TransportDelay  DelayTime=.001
  Clock : Clock
      settings: Decimation=10
  Latch1 : Subsystem  mask(Latch){@1=0}
      mask prompts: @1 "Initial State for Output "Q":"
      mask help: Latch
      mask init:
      | ini=(@1~=0);
      mask Help: Latches the S input.  When S (set) is one, the Q output  becomes one.  The output remains one until the R (reset) input becomes one, forcing the output to zero.  If both R and S are one, the latch will be in an undefined state.
      mask Display: disp('S   Q\n\nR  !Q')
  Logical Operator : Logic  Operator=OR  Inputs=3
  Logical Operator1 : Logic
  Logical Operator2 : Logic
  Relational Operator : RelationalOperator  InputSameDT=on
  SampHold?1 : Subsystem
      mask Display: disp('S&H\n(S=L)\n(H=H)')
  Sum : Sum  Inputs=+-  SaturateOnIntegerOverflow=on  InputSameDT=on
  event resettable? : Constant  Orientation=up
  leading edge detect : Subsystem
      mask Display: disp('Leading\nEdge Det')
  loop breaker : Memory  Orientation=left
  trailing edge detect : Subsystem
      mask Display: disp('Trailing\nEdge Det')
  out_1 : Outport  InitialOutput=0
  wires:
  event resettable?/1 -> Logical Operator2/2, Logical Operator1/2
  leading edge detect/1(out_1) -> Logical Operator2/1
  Logical Operator2/1 -> Logical Operator/2
  trailing edge detect/1(out_1) -> Logical Operator1/1, 1 msec/1
  Logical Operator1/1 -> Logical Operator/1
  loop breaker/1 -> Logical Operator/3
  _PG/1 -> leading edge detect/1(in_1), trailing edge detect/1(in_1)
  Latch1/1(out_1) -> SampHold?1/2(S/H?)
  Relational Operator/1 -> out_1/1, loop breaker/1
  Sum/1 -> Relational Operator/1
  Clock/1 -> Sum/1, SampHold?1/1(Input)
  SampHold?1/1(output) -> Sum/2
  Logical Operator/1 -> Latch1/2(in_2)
  1 msec/1 -> Latch1/1(in_1)
  _timer value (port)/1 -> Relational Operator/2

== system testtemp/BS Enable1/BS Timing/leading edge detect ==
  note: leading edge detection
  in_1 : Inport  Port=1  LatchInput=off
  Abs : Abs  SaturateOnIntegerOverflow=on
  Derivative : Derivative
  Relational Operator : RelationalOperator  Operator===  InputSameDT=on
  Sign : Subsystem
      mask Type: Sign
      mask Description: y = sign(x)
      mask Help: Sign Function:\n\t\t\ty = 1 if x > 0\n\t\t\ty = 0 if x = 0\n\t\t\ty = -1 if x < 0
      mask Display: plot(-50,-50,50,50,[-50,50],[0,0],[0,0],[-50,50],[-40,0],[-30,-30],[0,40],[30,30])
  Threshold 1 : Constant
  out_1 : Outport  InitialOutput=0
  wires:
  in_1/1 -> Abs/1
  Relational Operator/1 -> out_1/1
  Threshold 1/1 -> Relational Operator/2
  Sign/1(out_1) -> Relational Operator/1
  Derivative/1 -> Sign/1(in_1)
  Abs/1 -> Derivative/1

== system testtemp/PG+NI->OMN ->Plant/OMN/SampHold? ==
  note: When "S/H?" is LOW, then "Input" is switched directly to the
      | output ("sample").  When "S/H?" is HIGH, the current output is
      | maintained ("hold").
  Input : Inport  Port=1  LatchInput=off
  S/H? : Inport  Port=2  LatchInput=off
  Memory : Memory  Orientation=left
  Sign : Subsystem
      mask Type: Sign
      mask Description: y = sign(x)
      mask Help: Sign Function:\n\t\t\ty = 1 if x > 0\n\t\t\ty = 0 if x = 0\n\t\t\ty = -1 if x < 0
      mask Display: plot(-50,-50,50,50,[-50,50],[0,0],[0,0],[-50,50],[-40,0],[-30,-30],[0,40],[30,30])
  Switch2 : Switch  Threshold=0.5  SaturateOnIntegerOverflow=on  InputSameDT=on
  output : Outport  InitialOutput=0
  wires:
  Input/1 -> Switch2/3
  Memory/1 -> Switch2/1
  S/H?/1 -> Sign/1(in_1)
  Sign/1(out_1) -> Switch2/2
  Switch2/1 -> output/1, Memory/1

== system testtemp/PG+NI->OMN ->Plant/OMN/Sign ==
  in_1 : Inport  Port=1  LatchInput=off
  Constant : Constant  Value=0
  Relational Operator : RelationalOperator  Operator=>  InputSameDT=on
  Relational Operator1 : RelationalOperator  Operator=<  InputSameDT=on
  Sum : Sum  Inputs=+-  SaturateOnIntegerOverflow=on  InputSameDT=on
  out_1 : Outport  InitialOutput=0
  wires:
  Sum/1 -> out_1/1
  Relational Operator/1 -> Sum/1
  Relational Operator1/1 -> Sum/2
  Constant/1 -> Relational Operator1/2, Relational Operator/2
  in_1/1 -> Relational Operator/1, Relational Operator1/1

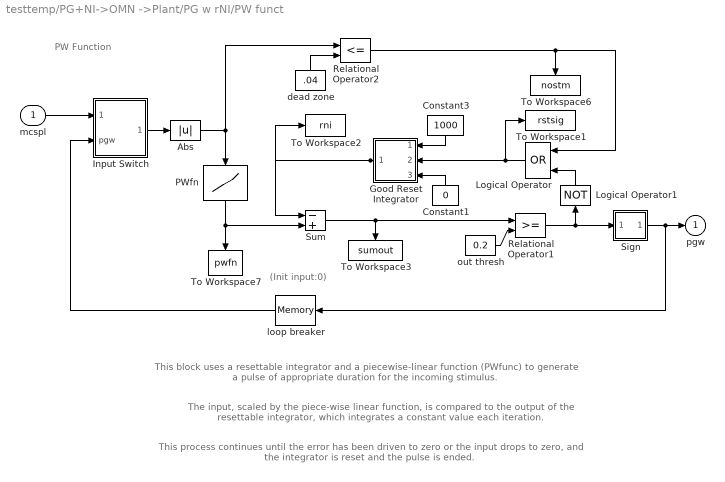
== system testtemp/PG+NI->OMN ->Plant/PG w rNI/PW funct ==
  note: PW Function
  note: (Init input:0)
  note: This block uses a resettable integrator and a piecewise-linear function (PWfunc) to generate
      | a pulse of appropriate duration for the incoming stimulus.
  note: The input, scaled by the piece-wise linear function, is compared to the output of the
      | resettable integrator, which integrates a constant value each iteration.
  note: This process continues until the error has been driven to zero or the input drops to zero,
      | and the integrator is reset and the pulse is ended.
  mcspl : Inport  Port=1  LatchInput=off
  Abs : Abs  SaturateOnIntegerOverflow=on
  Constant1 : Constant  Orientation=up  Value=0
  Constant3 : Constant  Orientation=down  Value=1000
  Good Reset Integrator : Subsystem  Orientation=left
      mask Display: disp('1/s')
  Input Switch : Subsystem
      mask Display: disp('Input\nSwitch')
  Logical Operator : Logic  Orientation=left  Operator=OR
  Logical Operator1 : Logic  Orientation=up  Operator=NOT  Inputs=1
  PWfn : Lookup  Orientation=down  InputValues=[ 0, 0.1:5, 5:10, 10:50 ]  OutputValues="[ 0, (0.1:5)*0+15,  (5:10)*1+10,  (10:50)*2]"  SaturateOnIntegerOverflow=on
  Relational Operator1 : RelationalOperator  InputSameDT=on
  Relational Operator2 : RelationalOperator  Operator=<=  InputSameDT=on
  Sign : Subsystem
      mask Type: Sign
      mask Description: y = sign(x)
      mask Help: Sign Function:\n\t\t\ty = 1 if x > 0\n\t\t\ty = 0 if x = 0\n\t\t\ty = -1 if x < 0
      mask Display: plot(-50,-50,50,50,[-50,50],[0,0],[0,0],[-50,50],[-40,0],[-30,-30],[0,40],[30,30])
  Sum : Sum  Inputs=-+  SaturateOnIntegerOverflow=on  InputSameDT=on
  To Workspace1 : ToWorkspace  VariableName=rstsig  SaveFormat=Array
      settings: MaxDataPoints=10000
  To Workspace2 : ToWorkspace  VariableName=rni  SaveFormat=Array
      settings: MaxDataPoints=10000
  To Workspace3 : ToWorkspace  VariableName=sumout  SaveFormat=Array
      settings: Orientation=down  MaxDataPoints=10000
  To Workspace6 : ToWorkspace  VariableName=nostm  SaveFormat=Array
      settings: Orientation=down  MaxDataPoints=10000
  To Workspace7 : ToWorkspace  VariableName=pwfn  SaveFormat=Array
      settings: Orientation=down  MaxDataPoints=10000
  dead zone : Constant  Orientation=up  Value=.04
  loop breaker : Memory  Orientation=left
  out thresh : Constant  Value=0.2
  pgw : Outport  InitialOutput=0
  wires:
  Abs/1 -> PWfn/1, Relational Operator2/1
  PWfn/1 -> To Workspace7/1, Sum/2
  Sign/1(out_1) -> pgw/1, loop breaker/1
  loop breaker/1 -> Input Switch/2(pgw)
  mcspl/1 -> Input Switch/1(mcspl)
  Input Switch/1(mcsw) -> Abs/1
  Sum/1 -> Relational Operator1/1, To Workspace3/1
  Logical Operator/1 -> Good Reset Integrator/2(in_2), To Workspace1/1
  Good Reset Integrator/1(out_1) -> Sum/1, To Workspace2/1
  Relational Operator2/1 -> To Workspace6/1, Logical Operator/1
  dead zone/1 -> Relational Operator2/2
  out thresh/1 -> Relational Operator1/2
  Constant1/1 -> Good Reset Integrator/3(in_3)
  Constant3/1 -> Good Reset Integrator/1(in_1)
  Relational Operator1/1 -> Logical Operator1/1, Sign/1(in_1)
  Logical Operator1/1 -> Logical Operator/2

== system testtemp/PG+NI->OMN ->Plant/PG w rNI/RefLatch (good) ==
  note: The "NOT" gate outputs a DISABLE signal whenever there is any
      | input, so that there can be no response.
  note: By ANDing these outputs, we get a signal that is DISABLED
      | starting with the beginning of the input pulse, and remains so until
      | rp milliseconds after the termination of the pulse.
  note: The falling edge" block's output becomes DISABLED upon
      | detection of the END of the input pulse, and remains
      | so until the refractory period of rp milliseconds has elapsed.
  note: It's a cheap trick, but it seems to work:
  in_1 : Inport  Port=1  LatchInput=off
  Abs : Abs  SaturateOnIntegerOverflow=on
  Logical Operator : Logic
  Logical Operator1 : Logic  Operator=NOT  Inputs=1
  trailing edge : Subsystem
      mask Display: disp('Refract\nLatch (te)')
  out_1 : Outport  InitialOutput=0
  wires:
  in_1/1 -> Abs/1
  Abs/1 -> Logical Operator1/1, trailing edge/1(in_1)
  trailing edge/1(out_1) -> Logical Operator/2
  Logical Operator1/1 -> Logical Operator/1
  Logical Operator/1 -> out_1/1

== system testtemp/PG+NI->OMN ->Plant/PG w rNI/SampHold?1 ==
  note: When "S/H?" is HIGH, then "Input" is switched directly to the
      | output ("sample").  When "S/H?" is LOW, the current output is
      | maintained ("hold").
  Input : Inport  Port=1  LatchInput=off
  S/H? : Inport  Port=2  LatchInput=off
  Memory : Memory  Orientation=left
  Sign : Subsystem
      mask Type: Sign
      mask Description: y = sign(x)
      mask Help: Sign Function:\n\t\t\ty = 1 if x > 0\n\t\t\ty = 0 if x = 0\n\t\t\ty = -1 if x < 0
      mask Display: plot(-50,-50,50,50,[-50,50],[0,0],[0,0],[-50,50],[-40,0],[-30,-30],[0,40],[30,30])
  Switch2 : Switch  Threshold=0.5  SaturateOnIntegerOverflow=on  InputSameDT=on
  output : Outport  InitialOutput=0
  wires:
  Memory/1 -> Switch2/3
  Input/1 -> Switch2/1
  Switch2/1 -> Memory/1, output/1
  Sign/1(out_1) -> Switch2/2
  S/H?/1 -> Sign/1(in_1)

== system testtemp/Pulse+NI-> OMN->Plant/OMN/SampHold? ==
  note: When "S/H?" is LOW, then "Input" is switched directly to the
      | output ("sample").  When "S/H?" is HIGH, the current output is
      | maintained ("hold").
  Input : Inport  Port=1  LatchInput=off
  S/H? : Inport  Port=2  LatchInput=off
  Memory : Memory  Orientation=left
  Sign : Subsystem
      mask Type: Sign
      mask Description: y = sign(x)
      mask Help: Sign Function:\n\t\t\ty = 1 if x > 0\n\t\t\ty = 0 if x = 0\n\t\t\ty = -1 if x < 0
      mask Display: plot(-50,-50,50,50,[-50,50],[0,0],[0,0],[-50,50],[-40,0],[-30,-30],[0,40],[30,30])
  Switch2 : Switch  Threshold=0.5  SaturateOnIntegerOverflow=on  InputSameDT=on
  output : Outport  InitialOutput=0
  wires:
  Input/1 -> Switch2/3
  Memory/1 -> Switch2/1
  S/H?/1 -> Sign/1(in_1)
  Sign/1(out_1) -> Switch2/2
  Switch2/1 -> output/1, Memory/1

== system testtemp/Pulse+NI-> OMN->Plant/OMN/Sign ==
  in_1 : Inport  Port=1  LatchInput=off
  Constant : Constant  Value=0
  Relational Operator : RelationalOperator  Operator=>  InputSameDT=on
  Relational Operator1 : RelationalOperator  Operator=<  InputSameDT=on
  Sum : Sum  Inputs=+-  SaturateOnIntegerOverflow=on  InputSameDT=on
  out_1 : Outport  InitialOutput=0
  wires:
  Sum/1 -> out_1/1
  Relational Operator/1 -> Sum/1
  Relational Operator1/1 -> Sum/2
  Constant/1 -> Relational Operator1/2, Relational Operator/2
  in_1/1 -> Relational Operator/1, Relational Operator1/1

== system testtemp/Target Velocity Reconstruction/SampHold?2/Sign ==
  in_1 : Inport  Port=1  LatchInput=off
  Constant : Constant  Value=0
  Relational Operator : RelationalOperator  Operator=>  InputSameDT=on
  Relational Operator1 : RelationalOperator  Operator=<  InputSameDT=on
  Sum : Sum  Inputs=+-  SaturateOnIntegerOverflow=on  InputSameDT=on
  out_1 : Outport  InitialOutput=0
  wires:
  in_1/1 -> Relational Operator/1, Relational Operator1/1
  Constant/1 -> Relational Operator1/2, Relational Operator/2
  Relational Operator1/1 -> Sum/2
  Relational Operator/1 -> Sum/1
  Sum/1 -> out_1/1

== system testtemp/Target Velocity Reconstruction/SampHold?4/Sign ==
  in_1 : Inport  Port=1  LatchInput=off
  Constant : Constant  Value=0
  Relational Operator : RelationalOperator  Operator=>  InputSameDT=on
  Relational Operator1 : RelationalOperator  Operator=<  InputSameDT=on
  Sum : Sum  Inputs=+-  SaturateOnIntegerOverflow=on  InputSameDT=on
  out_1 : Outport  InitialOutput=0
  wires:
  Sum/1 -> out_1/1
  Relational Operator/1 -> Sum/1
  Relational Operator1/1 -> Sum/2
  Constant/1 -> Relational Operator/2, Relational Operator1/2
  in_1/1 -> Relational Operator1/1, Relational Operator/1
